simulink model "three_phase_solar_grid_SSC"  (R2025b)
settings: Solver=VariableStepAuto  StartTime=0.0  StopTime=0.8  RelTol=1e-6
libraries: ee_lib x15, nesl_utility x13, fl_lib x10, simulink x3, eeTransforms x2, eeSinusoidalMeasurementV2 x1
settings Model: SimulationMode=accelerator  Creator=a6039  LastModifiedBy=agarcian
settings SolverCC: AlgebraicLoopSolver=TrustRegion
settings DebuggingCC: UnconnectedInputMsg=warning  UnconnectedOutputMsg=warning  UnconnectedLineMsg=warning
settings ModelReferenceCC: EnableRefExpFcnMdlSchedulingChecks=on
settings RTWCC: GPUComputeCapability=3.5  DLArmComputeVersion=19.05

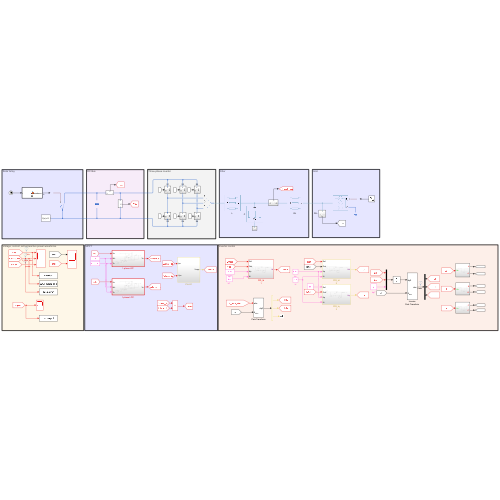
[thumbnail: Simulink's stored preview of the top-level diagram]
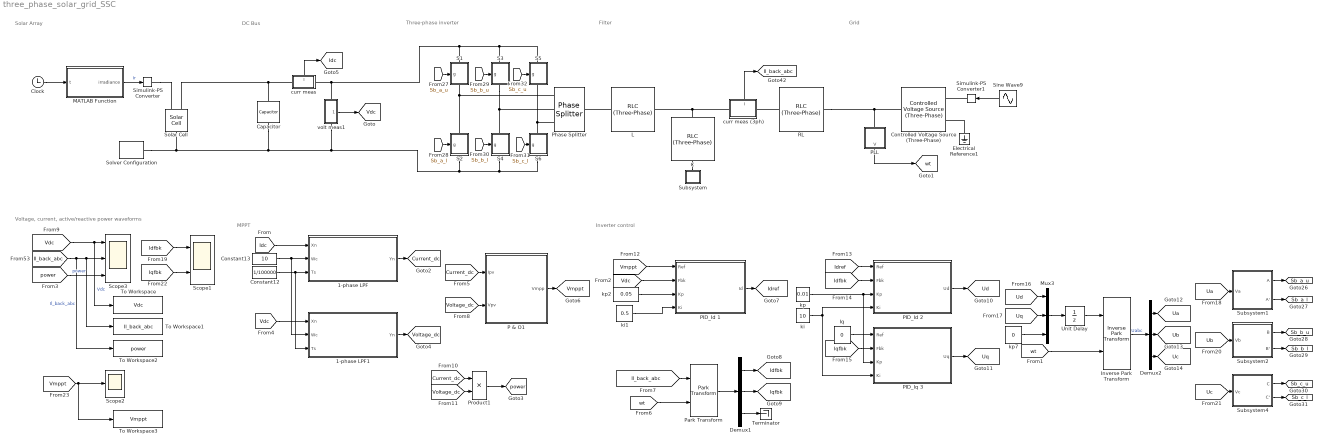
== system three_phase_solar_grid_SSC ==
  note: Filter
  note: Solar Array
  note: MPPT
  note: Three-phase inverter
  note: Inverter control
  note: Voltage, current, active/reactive power waveforms
  note: DC Bus
  note: Grid
  1-phase LPF : Subsystem  TreatAsAtomicUnit=on
  1-phase LPF1 : Subsystem  TreatAsAtomicUnit=on
  C : ee_lib/Passive/RLC Assemblies/RLC (Three-Phase)  port_option=ee.enum.threePhasePort.composite  component_structure=ee.enum.rlc.structure.C  R=1 Ohm  L=1e-3 H  C=1e-4 F  R_parasitic=0 Ohm  G_parasitic=0 1/Ohm  IL_specify=off  IL_priority=High  IL=[0, 0, 0] A  IL_nominal_specify=off  IL_nominal_value=1  IL_nominal_unit=A  VC_specify=off  VC_priority=High  VC=[0, 0, 0] V  VC_nominal_specify=off  VC_nominal_value=1  VC_nominal_unit=V
      settings: InternalSimscapePortConfiguration="{\"Bottom\":[],\"Left\":[{\"id\":\"N1\",\"label\":\"~1\",\"type\":\"foundation.electrical.three_phase\"}],\"Right\":[{\"id\":\"N2\",\"label\":\"~2\",\"type\":\"foundation.electrical.three_phase\"}],\"Top\":[]}"
  Capacitor : fl_lib/Electrical/Electrical Elements/Capacitor  c=1e-3 F  r=1e-8 Ohm  g=0 1/Ohm  i_specify=off  i_priority=None  i=0 A  i_nominal_specify=off  i_nominal_value=1  i_nominal_unit=A  v_specify=off  v_priority=None  v=0 V  v_nominal_specify=off  v_nominal_value=1  v_nominal_unit=V  vc_specify=off  vc_priority=High  vc=0 V  vc_nominal_specify=off  vc_nominal_value=1  vc_nominal_unit=V
  Clock : Clock
  Constant12 : Constant  Value=1/100000
  Constant13 : Constant  Value=10
  Controlled Voltage Source (Three-Phase) : ee_lib/Sources/Controlled Voltage Source (Three-Phase)  input_option=ee.enum.inputType.instantaneous  FRated=60 Hz
      settings: InternalSimscapePortConfiguration="{\"Bottom\":[],\"Left\":[{\"id\":\"S\",\"label\":\"S\",\"type\":\"input\"},{\"id\":\"n\",\"label\":\"n\",\"type\":\"foundation.electrical.electrical\"}],\"Right\":[{\"id\":\"N\",\"label\":\"~\",\"type\":\"foundation.electrical.three_phase\"}],\"Top\":[]}"
  Demux1 : Demux  Outputs=3
  Demux2 : Demux  Outputs=3
  Electrical Reference1 : fl_lib/Electrical/Electrical Elements/Electrical Reference
  Inverse Park Transform : eeTransforms/Inverse Park Transform  AxisAlignment=D-axis  PowerInvariant=off
      settings: LibrarySourceBlock=|
      | ee_sl_lib/Mathematical
      | Transforms/Inverse
      | Park Transform
  Iq : Constant  Value=0
  L : ee_lib/Passive/RLC Assemblies/RLC (Three-Phase)  port_option=ee.enum.threePhasePort.composite  component_structure=ee.enum.rlc.structure.L  R=1 Ohm  L=1e-3 H  C=1e-6 F  R_parasitic=0 Ohm  G_parasitic=0 1/Ohm  IL_specify=off  IL_priority=High  IL=[0, 0, 0] A  IL_nominal_specify=off  IL_nominal_value=1  IL_nominal_unit=A  VC_specify=off  VC_priority=High  VC=[0, 0, 0] V  VC_nominal_specify=off  VC_nominal_value=1  VC_nominal_unit=V
      settings: InternalSimscapePortConfiguration="{\"Bottom\":[],\"Left\":[{\"id\":\"N1\",\"label\":\"~1\",\"type\":\"foundation.electrical.three_phase\"}],\"Right\":[{\"id\":\"N2\",\"label\":\"~2\",\"type\":\"foundation.electrical.three_phase\"}],\"Top\":[]}"
  MATLAB Function : MATLAB Function  TreatAsAtomicUnit=on
  Mux3 : Mux  Inputs=3
  P & O1 : Subsystem
  PID_Id 1 : Subsystem
  PID_Id 2 : Subsystem
  PID_Iq 3 : Subsystem
  PLL : Subsystem
  Park Transform : eeTransforms/Park Transform  AxisAlignment=D-axis  PowerInvariant=off
      settings: LibrarySourceBlock=|
      | ee_sl_lib/Mathematical
      | Transforms/Park Transform
  Phase Splitter : ee_lib/Connectors & References/Phase Splitter
  Product1 : Product
  RL : ee_lib/Passive/RLC Assemblies/RLC (Three-Phase)  port_option=ee.enum.threePhasePort.composite  component_structure=ee.enum.rlc.structure.SeriesRL  R=0.1 Ohm  L=1e-9 H  C=1e-6 F  R_parasitic=0 Ohm  G_parasitic=0 1/Ohm  IL_specify=off  IL_priority=High  IL=[0, 0, 0] A  IL_nominal_specify=off  IL_nominal_value=1  IL_nominal_unit=A  VC_specify=off  VC_priority=High  VC=[0, 0, 0] V  VC_nominal_specify=off  VC_nominal_value=1  VC_nominal_unit=V
      settings: InternalSimscapePortConfiguration="{\"Bottom\":[],\"Left\":[{\"id\":\"N1\",\"label\":\"~1\",\"type\":\"foundation.electrical.three_phase\"}],\"Right\":[{\"id\":\"N2\",\"label\":\"~2\",\"type\":\"foundation.electrical.three_phase\"}],\"Top\":[]}"
  S1 : Subsystem
      settings: PortSchema="{\"entries\":[{\"content\":{\"sides\":[{\"content\":{\"connectorIds\":[\"In1\"]},\"type\":\"ConnectorPlacement.EquallySpacedRectSide\",\"uuid\":\"60fc8352-b056-4a1d-84e9-807da1ce3c88\"},{\"content\":{\"side\":\"RIGHT\"},\"type\":\"ConnectorPlacement.EquallySpacedRectSide\",\"uuid\":\"4f85bb6a-64c7-4bda-b651-7e84ba390faf\"},{\"content\":{\"connectorIds\":[\"LConn1\"],\"side\":\"TOP\"},\"type\":\"ConnectorPlacement.EquallySpacedRectSide\",\"uuid\":\"49a2dfe1-7dda-4371-a15a-7ad00d7eb6fd\"},{\"content\":{\"connectorIds\":[\"RConn1\"],\"side\":\"BOTTOM\"},\"type\":\"ConnectorPlacement.EquallySpacedRectSide\",\"uuid\":\"2b076144-f23a-4c54-b109-69957c2c042c\"}]},\"type\":\"ConnectorPlacement.EquallySpacedConnector\",\"uuid\":\"c494b7b1-a248-4760-aec7-aedba1239c75\"}],\"packageUris\":[\"http://schema.mathworks.com/mf0/Connector/R2020b\"],\"version\":\"1.0\"}"
  S2 : Subsystem
      settings: PortSchema="{\"entries\":[{\"content\":{\"sides\":[{\"content\":{\"connectorIds\":[\"In1\"]},\"type\":\"ConnectorPlacement.EquallySpacedRectSide\",\"uuid\":\"60fc8352-b056-4a1d-84e9-807da1ce3c88\"},{\"content\":{\"side\":\"RIGHT\"},\"type\":\"ConnectorPlacement.EquallySpacedRectSide\",\"uuid\":\"4f85bb6a-64c7-4bda-b651-7e84ba390faf\"},{\"content\":{\"connectorIds\":[\"LConn1\"],\"side\":\"TOP\"},\"type\":\"ConnectorPlacement.EquallySpacedRectSide\",\"uuid\":\"49a2dfe1-7dda-4371-a15a-7ad00d7eb6fd\"},{\"content\":{\"connectorIds\":[\"RConn1\"],\"side\":\"BOTTOM\"},\"type\":\"ConnectorPlacement.EquallySpacedRectSide\",\"uuid\":\"2b076144-f23a-4c54-b109-69957c2c042c\"}]},\"type\":\"ConnectorPlacement.EquallySpacedConnector\",\"uuid\":\"c494b7b1-a248-4760-aec7-aedba1239c75\"}],\"packageUris\":[\"http://schema.mathworks.com/mf0/Connector/R2020b\"],\"version\":\"1.0\"}"
  S3 : Subsystem
      settings: PortSchema="{\"entries\":[{\"content\":{\"sides\":[{\"content\":{\"connectorIds\":[\"In1\"]},\"type\":\"ConnectorPlacement.EquallySpacedRectSide\",\"uuid\":\"60fc8352-b056-4a1d-84e9-807da1ce3c88\"},{\"content\":{\"side\":\"RIGHT\"},\"type\":\"ConnectorPlacement.EquallySpacedRectSide\",\"uuid\":\"4f85bb6a-64c7-4bda-b651-7e84ba390faf\"},{\"content\":{\"connectorIds\":[\"LConn1\"],\"side\":\"TOP\"},\"type\":\"ConnectorPlacement.EquallySpacedRectSide\",\"uuid\":\"49a2dfe1-7dda-4371-a15a-7ad00d7eb6fd\"},{\"content\":{\"connectorIds\":[\"RConn1\"],\"side\":\"BOTTOM\"},\"type\":\"ConnectorPlacement.EquallySpacedRectSide\",\"uuid\":\"2b076144-f23a-4c54-b109-69957c2c042c\"}]},\"type\":\"ConnectorPlacement.EquallySpacedConnector\",\"uuid\":\"c494b7b1-a248-4760-aec7-aedba1239c75\"}],\"packageUris\":[\"http://schema.mathworks.com/mf0/Connector/R2020b\"],\"version\":\"1.0\"}"
  S4 : Subsystem
      settings: PortSchema="{\"entries\":[{\"content\":{\"sides\":[{\"content\":{\"connectorIds\":[\"In1\"]},\"type\":\"ConnectorPlacement.EquallySpacedRectSide\",\"uuid\":\"60fc8352-b056-4a1d-84e9-807da1ce3c88\"},{\"content\":{\"side\":\"RIGHT\"},\"type\":\"ConnectorPlacement.EquallySpacedRectSide\",\"uuid\":\"4f85bb6a-64c7-4bda-b651-7e84ba390faf\"},{\"content\":{\"connectorIds\":[\"LConn1\"],\"side\":\"TOP\"},\"type\":\"ConnectorPlacement.EquallySpacedRectSide\",\"uuid\":\"49a2dfe1-7dda-4371-a15a-7ad00d7eb6fd\"},{\"content\":{\"connectorIds\":[\"RConn1\"],\"side\":\"BOTTOM\"},\"type\":\"ConnectorPlacement.EquallySpacedRectSide\",\"uuid\":\"2b076144-f23a-4c54-b109-69957c2c042c\"}]},\"type\":\"ConnectorPlacement.EquallySpacedConnector\",\"uuid\":\"c494b7b1-a248-4760-aec7-aedba1239c75\"}],\"packageUris\":[\"http://schema.mathworks.com/mf0/Connector/R2020b\"],\"version\":\"1.0\"}"
  S5 : Subsystem
      settings: PortSchema="{\"entries\":[{\"content\":{\"sides\":[{\"content\":{\"connectorIds\":[\"In1\"]},\"type\":\"ConnectorPlacement.EquallySpacedRectSide\",\"uuid\":\"60fc8352-b056-4a1d-84e9-807da1ce3c88\"},{\"content\":{\"side\":\"RIGHT\"},\"type\":\"ConnectorPlacement.EquallySpacedRectSide\",\"uuid\":\"4f85bb6a-64c7-4bda-b651-7e84ba390faf\"},{\"content\":{\"connectorIds\":[\"LConn1\"],\"side\":\"TOP\"},\"type\":\"ConnectorPlacement.EquallySpacedRectSide\",\"uuid\":\"49a2dfe1-7dda-4371-a15a-7ad00d7eb6fd\"},{\"content\":{\"connectorIds\":[\"RConn1\"],\"side\":\"BOTTOM\"},\"type\":\"ConnectorPlacement.EquallySpacedRectSide\",\"uuid\":\"2b076144-f23a-4c54-b109-69957c2c042c\"}]},\"type\":\"ConnectorPlacement.EquallySpacedConnector\",\"uuid\":\"c494b7b1-a248-4760-aec7-aedba1239c75\"}],\"packageUris\":[\"http://schema.mathworks.com/mf0/Connector/R2020b\"],\"version\":\"1.0\"}"
  S6 : Subsystem
      settings: PortSchema="{\"entries\":[{\"content\":{\"sides\":[{\"content\":{\"connectorIds\":[\"In1\"]},\"type\":\"ConnectorPlacement.EquallySpacedRectSide\",\"uuid\":\"60fc8352-b056-4a1d-84e9-807da1ce3c88\"},{\"content\":{\"side\":\"RIGHT\"},\"type\":\"ConnectorPlacement.EquallySpacedRectSide\",\"uuid\":\"4f85bb6a-64c7-4bda-b651-7e84ba390faf\"},{\"content\":{\"connectorIds\":[\"LConn1\"],\"side\":\"TOP\"},\"type\":\"ConnectorPlacement.EquallySpacedRectSide\",\"uuid\":\"49a2dfe1-7dda-4371-a15a-7ad00d7eb6fd\"},{\"content\":{\"connectorIds\":[\"RConn1\"],\"side\":\"BOTTOM\"},\"type\":\"ConnectorPlacement.EquallySpacedRectSide\",\"uuid\":\"2b076144-f23a-4c54-b109-69957c2c042c\"}]},\"type\":\"ConnectorPlacement.EquallySpacedConnector\",\"uuid\":\"c494b7b1-a248-4760-aec7-aedba1239c75\"}],\"packageUris\":[\"http://schema.mathworks.com/mf0/Connector/R2020b\"],\"version\":\"1.0\"}"
  Scope1 : Scope  NumInputPorts=2
      settings: ActiveDisplayYMinimum=-149.18655  ActiveDisplayYMaximum=893.7115
  Scope2 : Scope
      settings: ActiveDisplayYMinimum=356.99125  ActiveDisplayYMaximum=407.77875  DataLoggingVariableName=ScopeData2
  Scope3 : Scope  NumInputPorts=3
      settings: ActiveDisplayYMinimum=-56.521329530696754  ActiveDisplayYMaximum=508.69198645627091  DataLoggingVariableName=ScopeData3
  Simulink-PS Converter : nesl_utility/Simulink-PS Converter  PhysicalDomain=network_engine_domain  SubClassName=ps_input  LeftPortType=input  RightPortType=output  PseudoPeriodic=off  Frequencies=[]  NoiseDistribution=none  NoiseParameters=[]  Unit=1  AffineConversion=off  FilteringAndDerivatives=provide  SimscapeFilterOrder=1  InputFilterTimeConstant=0.001  UdotUserProvided=0
  Simulink-PS Converter1 : nesl_utility/Simulink-PS Converter  PhysicalDomain=network_engine_domain  SubClassName=ps_input  LeftPortType=input  RightPortType=output  PseudoPeriodic=off  Frequencies=[]  NoiseDistribution=none  NoiseParameters=[]  Unit=1  AffineConversion=off  FilteringAndDerivatives=provide  SimscapeFilterOrder=1  InputFilterTimeConstant=0.001  UdotUserProvided=0
  Sine Wave9 : Sin  Amplitude=169.7  Frequency=60*2*pi  Phase=[0 -1 1]*2*pi/3  SampleTime=0
  Solar Cell : ee_lib/Sources/Solar Cell  prm=ee.enum.sources.solar_cell_prm.datasheet  Isc=5.17 A  Voc=43.99/72 V  Is=1e-6 A  Is2=0 A  Iph=7.34 A  Ir0=1000 W/m^2  ec=1.5  N2=2  Rs=0 Ohm  Rp=inf Ohm  N_series=10*72  N_parallel=40  TIPH1=0 1/K  EG=1.11 eV  TXIS1=3  TXIS2=3  TRS1=0  TRP1=0  Tmeas=25 degC  TFIXED=25 degC  thermal_mass=100 J/K  initial_temperature=25 degC
  Solver Configuration : nesl_utility/Solver Configuration  PhysicalDomain=network_engine_domain  SubClassName=solver  LeftPortType=input  RightPortType=generic  Tones=[]  Harmonics=[]  SimulateNoise=off  Profile=off  UseLocalSampling=off  EnableSwitchedLinearOptims=on  FrequencyDomain=off  UseCCode=off  RelTol=0.001  AbsTol=0.001  MinStep=1e-09  ToWorkspace=off  RevertToSquareIcSolve=off  NumHomotopyIterations=100  PhasorMode=off  PhasorModeNumHarmonics=1  ConsistencySolver=NEWTON_XTOL_AFTER_FTOL  IndexReductionMethod=DerivativeReplacement  DoDC=off  ResidualTolerance=1e-09  ConsistencyTolSource=GLOBAL  ConsistencyAbsTol=0.001  ConsistencyRelTol=0.001  ConsistencyTolFactor=0.001  UseLocalSolver=on  LocalSolverChoice=NE_BACKWARD_EULER_ADVANCER  ResolveIndetEquations=off  FunctionEvalNumThread=1  LocalSolverSampleTime=1e-7  DoFixedCost=on  MaxNonlinIter=2  MaxModeIter=2  ComputeImpulses=off  ImpulseIterations=2  LinearAlgebra=auto  LinearAlgebraNumThread=0  EquationFormulation=NE_TIME_EF  DelaysMemoryBudget=1024  AutomaticFiltering=off  FilteringTimeConstant=0.001  PartitionStorageMethod=AS_NEEDED  PartitionMemoryBudget=1024  PartitionMethod=FAST  MultibodyUseLocalSolver=off  MultibodyLocalSolverChoice=ODE1  MultibodyLocalSolverSampleTime=0.001
  Subsystem : Subsystem
  Subsystem1 : Subsystem
  Subsystem2 : Subsystem
  Subsystem4 : Subsystem
  Terminator : Terminator
  To Workspace : ToWorkspace  VariableName=Vdc  SaveFormat=Structure With Time  SampleTime=-1
  To Workspace1 : ToWorkspace  VariableName=Il_back_abc  SaveFormat=Structure With Time  SampleTime=-1
  To Workspace2 : ToWorkspace  VariableName=power  SaveFormat=Structure With Time  SampleTime=-1
  To Workspace3 : ToWorkspace  VariableName=Vmppt  SaveFormat=Structure With Time  SampleTime=-1
  Unit Delay : UnitDelay  SampleTime=-1  HasFrameUpgradeWarning=on
  curr meas : Subsystem
      settings: PortSchema="{\"entries\":[{\"content\":{\"sides\":[{\"content\":{\"connectorIds\":[\"LConn1\"]},\"type\":\"ConnectorPlacement.EquallySpacedRectSide\",\"uuid\":\"624dd8c9-1efa-425a-b23f-9e7d392e4567\"},{\"content\":{\"connectorIds\":[\"RConn1\"],\"side\":\"RIGHT\"},\"type\":\"ConnectorPlacement.EquallySpacedRectSide\",\"uuid\":\"c564bb74-22a6-4c48-884d-57ae53c7e586\"},{\"content\":{\"connectorIds\":[\"Out1\"],\"side\":\"TOP\"},\"type\":\"ConnectorPlacement.EquallySpacedRectSide\",\"uuid\":\"df3a0756-8bf4-4498-aa4e-0bb1b4f3eded\"}]},\"type\":\"ConnectorPlacement.EquallySpacedConnector\",\"uuid\":\"9eff73ec-b3ab-492c-96fa-8ca694a66385\"}],\"packageUris\":[\"http://schema.mathworks.com/mf0/Connector/R2020b\"],\"version\":\"1.0\"}"
  curr meas (3ph) : Subsystem
      settings: PortSchema="{\"entries\":[{\"content\":{\"sides\":[{\"content\":{\"connectorIds\":[\"LConn1\"]},\"type\":\"ConnectorPlacement.EquallySpacedRectSide\",\"uuid\":\"624dd8c9-1efa-425a-b23f-9e7d392e4567\"},{\"content\":{\"connectorIds\":[\"RConn1\"],\"side\":\"RIGHT\"},\"type\":\"ConnectorPlacement.EquallySpacedRectSide\",\"uuid\":\"c564bb74-22a6-4c48-884d-57ae53c7e586\"},{\"content\":{\"connectorIds\":[\"Out1\"],\"side\":\"TOP\"},\"type\":\"ConnectorPlacement.EquallySpacedRectSide\",\"uuid\":\"df3a0756-8bf4-4498-aa4e-0bb1b4f3eded\"}]},\"type\":\"ConnectorPlacement.EquallySpacedConnector\",\"uuid\":\"9eff73ec-b3ab-492c-96fa-8ca694a66385\"}],\"packageUris\":[\"http://schema.mathworks.com/mf0/Connector/R2020b\"],\"version\":\"1.0\"}"
  ki : Constant  Value=10
  ki1 : Constant  Value=0.5
  kp : Constant  Value=0.01
  kp2 : Constant  Value=0.05
  kp7 : Constant  Value=0
  volt meas1 : Subsystem
      settings: PortSchema="{\"entries\":[{\"content\":{\"sides\":[{\"content\":{},\"type\":\"ConnectorPlacement.EquallySpacedRectSide\",\"uuid\":\"624dd8c9-1efa-425a-b23f-9e7d392e4567\"},{\"content\":{\"connectorIds\":[\"Out1\"],\"side\":\"RIGHT\"},\"type\":\"ConnectorPlacement.EquallySpacedRectSide\",\"uuid\":\"c564bb74-22a6-4c48-884d-57ae53c7e586\"},{\"content\":{\"connectorIds\":[\"LConn1\"],\"side\":\"TOP\"},\"type\":\"ConnectorPlacement.EquallySpacedRectSide\",\"uuid\":\"df3a0756-8bf4-4498-aa4e-0bb1b4f3eded\"},{\"content\":{\"connectorIds\":[\"RConn1\"],\"side\":\"BOTTOM\"},\"type\":\"ConnectorPlacement.EquallySpacedRectSide\",\"uuid\":\"6b8e9540-8d6f-4bd3-bf1f-20eb25478a8e\"}]},\"type\":\"ConnectorPlacement.EquallySpacedConnector\",\"uuid\":\"9eff73ec-b3ab-492c-96fa-8ca694a66385\"}],\"packageUris\":[\"http://schema.mathworks.com/mf0/Connector/R2020b\"],\"version\":\"1.0\"}"
  tag scope: Current_dc=global, Idc=global, Idfbk=global, Idref=global, Il_back_abc=global, Iqfbk=global, Sb_a_l=global, Sb_a_u=global, Sb_b_l=global, Sb_b_u=global, Sb_c_l=global, Sb_c_u=global, Ua=global, Ub=global, Uc=global, Ud=global, Uq=global, Vdc=global, Vmppt=global, Voltage_dc=global, power=global, wt=global
  wires:
  [Il_back_abc] -> To Workspace2/1, To Workspace1/1, Scope3/2  "Il_back_abc"
  Iq/1 -> PID_Iq 3/1(Ref)
  Park Transform/1 -> Demux1/1
  [wt] -> Inverse Park Transform/2
  kp/1 -> PID_Iq 3/3(Kp), PID_Id 2/3(Kp)
  ki/1 -> PID_Id 2/4(Ki), PID_Iq 3/4(Ki)
  Mux3/1 -> Unit Delay/1
  [wt] -> Park Transform/2
  Inverse Park Transform/1 -> Demux2/1  "Uabc"
  [Il_back_abc] -> Park Transform/1
  [Sb_a_u] -> S1/1(g)
  [Sb_b_u] -> S3/1(g)
  [Sb_c_u] -> S5/1(g)
  [Sb_a_l] -> S2/1(g)
  [Sb_b_l] -> S4/1(g)
  [Sb_c_l] -> S6/1(g)
  volt meas1/1(V) -> [Vdc]
  [Vdc] -> PID_Id 1/2(Fbk)
  kp2/1 -> PID_Id 1/3(Kp)
  ki1/1 -> PID_Id 1/4(Ki)
  Constant12/1 -> 1-phase LPF1/3(Ts), 1-phase LPF/3(Ts)
  Constant13/1 -> 1-phase LPF1/2(Wc), 1-phase LPF/2(Wc)
  [Idc] -> 1-phase LPF/1(Xn)
  [Vdc] -> 1-phase LPF1/1(Xn)
  Subsystem1/1(A) -> [Sb_a_u]
  Subsystem1/2(A') -> [Sb_a_l]
  Subsystem2/1(B) -> [Sb_b_u]
  Subsystem2/2(B') -> [Sb_b_l]
  Subsystem4/1(C) -> [Sb_c_u]
  Subsystem4/2(C') -> [Sb_c_l]
  kp7/1 -> Mux3/3
  [Vdc] -> To Workspace/1, Scope3/1  "Vdc"
  [power] -> Scope3/3  "power"
  Product1/1 -> [power]
  Clock/1 -> MATLAB Function/1(t)
  1-phase LPF/1(Yn) -> [Current_dc]
  1-phase LPF1/1(Yn) -> [Voltage_dc]
  [Current_dc] -> P & O1/1(Ipv)
  [Voltage_dc] -> P & O1/2(Vpv)
  [Current_dc] -> Product1/1
  [Voltage_dc] -> Product1/2
  P & O1/1(Vmpp) -> [Vmppt]
  [Vmppt] -> PID_Id 1/1(Ref)
  PID_Id 1/1(Id) -> [Idref]
  [Idref] -> PID_Id 2/1(Ref)
  Demux1/1 -> [Idfbk]
  Demux1/2 -> [Iqfbk]
  [Idfbk] -> PID_Id 2/2(Fbk)
  [Iqfbk] -> PID_Iq 3/2(Fbk)
  PID_Id 2/1(Ud) -> [Ud]
  PID_Iq 3/1(Uq) -> [Uq]
  [Ud] -> Mux3/1
  [Uq] -> Mux3/2
  Demux2/1 -> [Ua]
  Demux2/2 -> [Ub]
  Demux2/3 -> [Uc]
  [Ua] -> Subsystem1/1(Va)
  [Ub] -> Subsystem2/1(Vb)
  [Uc] -> Subsystem4/1(Vc)
  [Idfbk] -> Scope1/1
  [Iqfbk] -> Scope1/2
  [Vmppt] -> To Workspace3/1, Scope2/1
  MATLAB Function/1(irradiance) -> Simulink-PS Converter/1  "Ir"
  curr meas/1(I) -> [Idc]
  curr meas (3ph)/1(I) -> [Il_back_abc]
  Sine Wave9/1 -> Simulink-PS Converter1/1
  Unit Delay/1 -> Inverse Park Transform/1
  Demux1/3 -> Terminator/1
  PLL/1(V) -> [wt]
  connections:
  volt meas1/LConn1 -- S5/LConn1 -- S3/LConn1 -- S1/LConn1 -- curr meas/RConn1
  Phase Splitter/RConn2 -- S3/RConn1 -- S4/LConn1
  Solver Configuration/RConn1 -- S6/RConn1 -- S4/RConn1 -- S2/RConn1 -- volt meas1/RConn1 -- Capacitor/RConn1 -- Solar Cell/RConn1
  Simulink-PS Converter/RConn1 -- Solar Cell/LConn1
  Phase Splitter/RConn1 -- S2/LConn1 -- S1/RConn1
  L/LConn1 -- Phase Splitter/LConn1
  C/LConn1 -- curr meas (3ph)/LConn1 -- L/RConn1
  RL/LConn1 -- curr meas (3ph)/RConn1
  RL/RConn1 -- Controlled Voltage Source (Three-Phase)/RConn1 -- PLL/LConn1
  Simulink-PS Converter1/RConn1 -- Controlled Voltage Source (Three-Phase)/LConn1
  Electrical Reference1/LConn1 -- Controlled Voltage Source (Three-Phase)/LConn2
  S6/LConn1 -- Phase Splitter/RConn3 -- S5/RConn1
  C/RConn1 -- Subsystem/LConn1
  Capacitor/LConn1 -- Solar Cell/LConn2 -- curr meas/LConn1

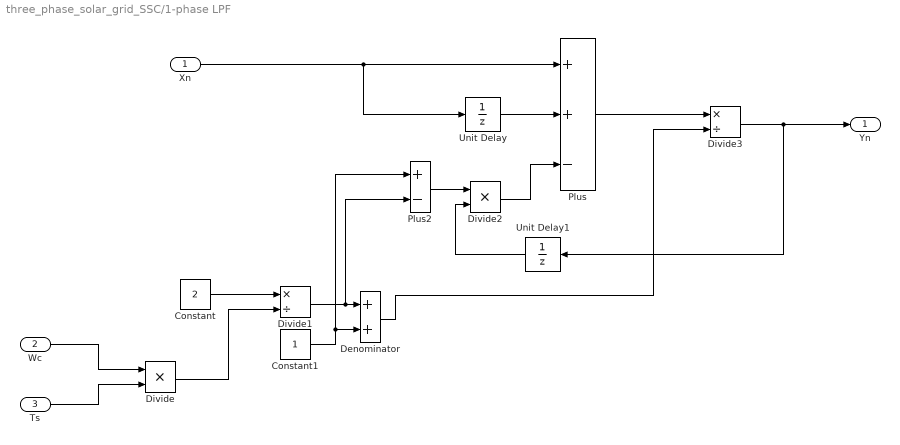
== system three_phase_solar_grid_SSC/1-phase LPF ==
  Xn : Inport
  Wc : Inport  Port=2
  Ts : Inport  Port=3
  Constant : Constant  Value=2
  Constant1 : Constant
  Denominator : Sum
  Divide : Product  Inputs=**
  Divide1 : Product  Inputs=*/
  Divide2 : Product  Inputs=**
  Divide3 : Product  Inputs=*/
  Plus : Sum  Inputs=++-
  Plus2 : Sum  Inputs=+-
  Unit Delay : UnitDelay  SampleTime=-1  HasFrameUpgradeWarning=on
  Unit Delay1 : UnitDelay  SampleTime=-1  HasFrameUpgradeWarning=on
  Yn : Outport
  wires:
  Xn/1 -> Unit Delay/1, Plus/1
  Unit Delay/1 -> Plus/2
  Wc/1 -> Divide/1
  Ts/1 -> Divide/2
  Divide/1 -> Divide1/2
  Constant/1 -> Divide1/1
  Divide1/1 -> Plus2/2, Denominator/1
  Constant1/1 -> Plus2/1, Denominator/2
  Plus2/1 -> Divide2/1
  Unit Delay1/1 -> Divide2/2
  Plus/1 -> Divide3/1
  Denominator/1 -> Divide3/2
  Divide3/1 -> Unit Delay1/1, Yn/1
  Divide2/1 -> Plus/3

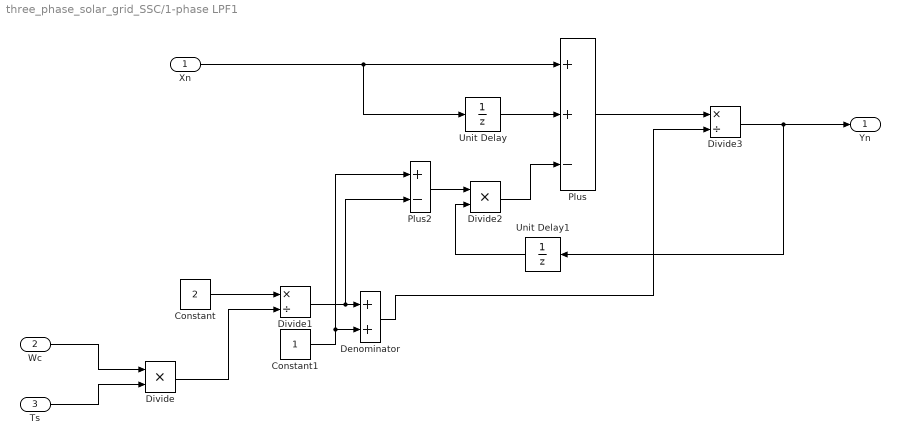
== system three_phase_solar_grid_SSC/1-phase LPF1 ==
  Xn : Inport
  Wc : Inport  Port=2
  Ts : Inport  Port=3
  Constant : Constant  Value=2
  Constant1 : Constant
  Denominator : Sum
  Divide : Product  Inputs=**
  Divide1 : Product  Inputs=*/
  Divide2 : Product  Inputs=**
  Divide3 : Product  Inputs=*/
  Plus : Sum  Inputs=++-
  Plus2 : Sum  Inputs=+-
  Unit Delay : UnitDelay  SampleTime=-1  HasFrameUpgradeWarning=on
  Unit Delay1 : UnitDelay  SampleTime=-1  HasFrameUpgradeWarning=on
  Yn : Outport
  wires:
  Xn/1 -> Unit Delay/1, Plus/1
  Unit Delay/1 -> Plus/2
  Wc/1 -> Divide/1
  Ts/1 -> Divide/2
  Divide/1 -> Divide1/2
  Constant/1 -> Divide1/1
  Divide1/1 -> Plus2/2, Denominator/1
  Constant1/1 -> Plus2/1, Denominator/2
  Plus2/1 -> Divide2/1
  Unit Delay1/1 -> Divide2/2
  Plus/1 -> Divide3/1
  Denominator/1 -> Divide3/2
  Divide3/1 -> Unit Delay1/1, Yn/1
  Divide2/1 -> Plus/3

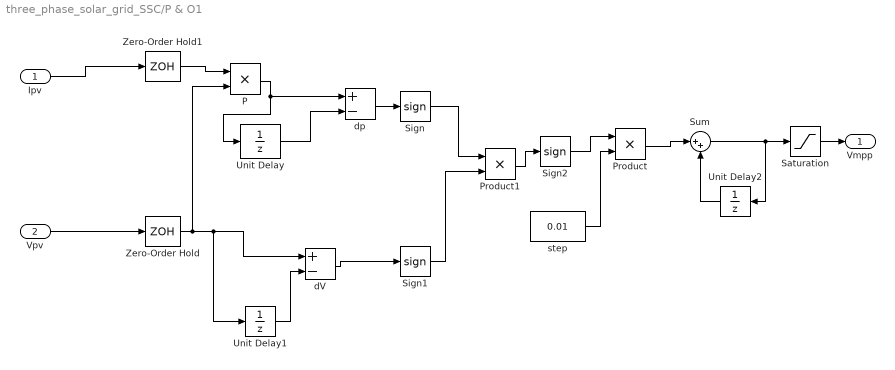
== system three_phase_solar_grid_SSC/P & O1 ==
  Ipv : Inport
  Vpv : Inport  Port=2
  P : Product  RndMeth=Zero
  Product : Product  RndMeth=Zero
  Product1 : Product  RndMeth=Zero
  Saturation : Saturate  UpperLimit=450  LowerLimit=0  LinearizeAsGain=off  ZeroCross=off
  Sign : Signum
  Sign1 : Signum
  Sign2 : Signum
  Sum : Sum  Inputs=|++
  Unit Delay : UnitDelay  SampleTime=-1  HasFrameUpgradeWarning=on
  Unit Delay1 : UnitDelay  SampleTime=-1  HasFrameUpgradeWarning=on
  Unit Delay2 : UnitDelay  InitialCondition=400  SampleTime=-1  HasFrameUpgradeWarning=on
  Zero-Order Hold : ZeroOrderHold  SampleTime=1/100000
  Zero-Order Hold1 : ZeroOrderHold  SampleTime=1/100000
  dV : Sum  Inputs=+-
  dp : Sum  Inputs=+-
  step : Constant  Value=0.01  SampleTime=1/100000
  Vmpp : Outport
  wires:
  Unit Delay1/1 -> dV/2
  Unit Delay/1 -> dp/2
  dV/1 -> Sign1/1
  step/1 -> Product/2
  Product/1 -> Sum/1
  Sign/1 -> Product1/1
  Sign1/1 -> Product1/2
  Product1/1 -> Sign2/1
  Ipv/1 -> Zero-Order Hold1/1
  Vpv/1 -> Zero-Order Hold/1
  P/1 -> Unit Delay/1, dp/1
  dp/1 -> Sign/1
  Sign2/1 -> Product/1
  Sum/1 -> Saturation/1, Unit Delay2/1
  Unit Delay2/1 -> Sum/2
  Zero-Order Hold/1 -> P/2, Unit Delay1/1, dV/1
  Zero-Order Hold1/1 -> P/1
  Saturation/1 -> Vmpp/1

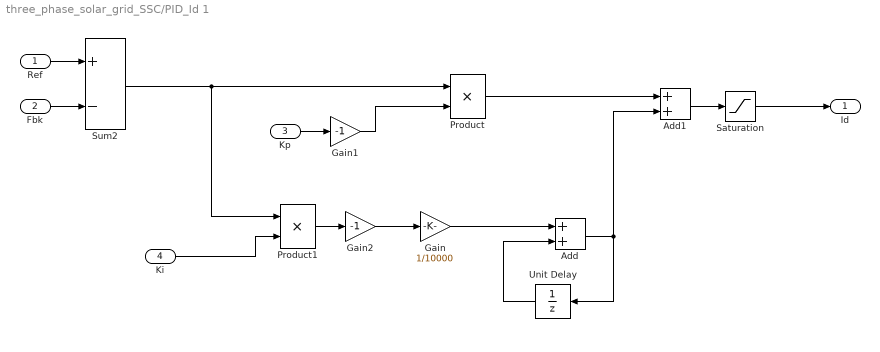
== system three_phase_solar_grid_SSC/PID_Id 1 ==
  Ref : Inport
  Fbk : Inport  Port=2
  Kp : Inport  Port=3
  Ki : Inport  Port=4
  Add : Sum
  Add1 : Sum
  Gain : Gain  Gain=1/10000
  Gain1 : Gain  Gain=-1
  Gain2 : Gain  Gain=-1
  Product : Product  OutDataTypeStr=Inherit: Same as first input
  Product1 : Product  OutDataTypeStr=Inherit: Same as first input
  Saturation : Saturate  UpperLimit=1000  LowerLimit=0  LinearizeAsGain=off  ZeroCross=off
  Sum2 : Sum  Inputs=+-
  Unit Delay : UnitDelay  SampleTime=-1  HasFrameUpgradeWarning=on
  Id : Outport
  wires:
  Sum2/1 -> Product1/1, Product/1
  Fbk/1 -> Sum2/2
  Ref/1 -> Sum2/1
  Product1/1 -> Gain2/1
  Add/1 -> Unit Delay/1, Add1/2
  Product/1 -> Add1/1
  Gain/1 -> Add/1
  Unit Delay/1 -> Add/2
  Kp/1 -> Gain1/1
  Ki/1 -> Product1/2
  Gain1/1 -> Product/2
  Gain2/1 -> Gain/1
  Add1/1 -> Saturation/1
  Saturation/1 -> Id/1

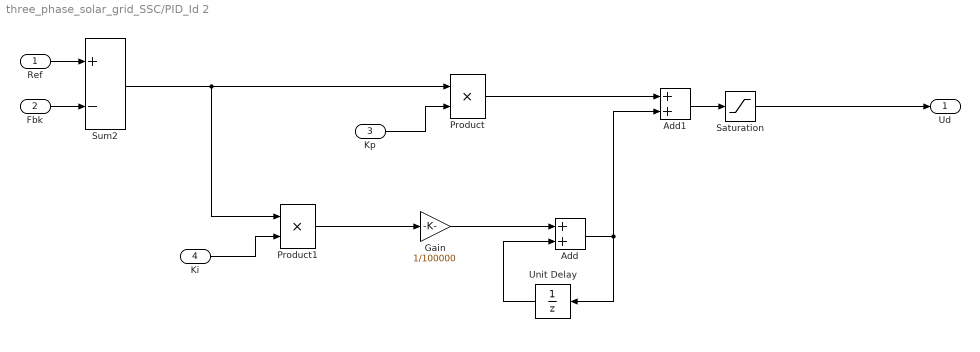
== system three_phase_solar_grid_SSC/PID_Id 2 ==
  Ref : Inport
  Fbk : Inport  Port=2
  Kp : Inport  Port=3
  Ki : Inport  Port=4
  Add : Sum
  Add1 : Sum
  Gain : Gain  Gain=1/100000
  Product : Product  OutDataTypeStr=Inherit: Same as first input
  Product1 : Product  OutDataTypeStr=Inherit: Same as first input
  Saturation : Saturate  UpperLimit=500  LowerLimit=-500  LinearizeAsGain=off  ZeroCross=off
  Sum2 : Sum  Inputs=+-
  Unit Delay : UnitDelay  InitialCondition=400  SampleTime=-1  HasFrameUpgradeWarning=on
  Ud : Outport
  wires:
  Add1/1 -> Saturation/1
  Sum2/1 -> Product1/1, Product/1
  Fbk/1 -> Sum2/2
  Ref/1 -> Sum2/1
  Kp/1 -> Product/2
  Ki/1 -> Product1/2
  Product1/1 -> Gain/1
  Add/1 -> Unit Delay/1, Add1/2
  Product/1 -> Add1/1
  Saturation/1 -> Ud/1
  Gain/1 -> Add/1
  Unit Delay/1 -> Add/2

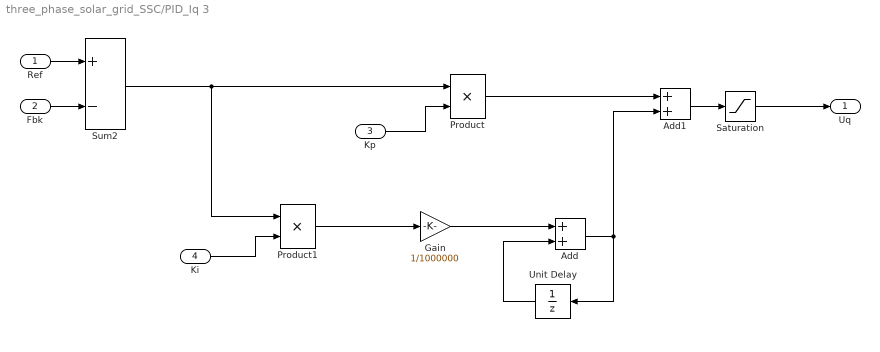
== system three_phase_solar_grid_SSC/PID_Iq 3 ==
  Ref : Inport
  Fbk : Inport  Port=2
  Kp : Inport  Port=3
  Ki : Inport  Port=4
  Add : Sum
  Add1 : Sum
  Gain : Gain  Gain=1/1000000
  Product : Product  OutDataTypeStr=Inherit: Same as first input
  Product1 : Product  OutDataTypeStr=Inherit: Same as first input
  Saturation : Saturate  UpperLimit=500  LowerLimit=-500  LinearizeAsGain=off  ZeroCross=off
  Sum2 : Sum  Inputs=+-
  Unit Delay : UnitDelay  SampleTime=-1  HasFrameUpgradeWarning=on
  Uq : Outport
  wires:
  Add1/1 -> Saturation/1
  Sum2/1 -> Product1/1, Product/1
  Fbk/1 -> Sum2/2
  Ref/1 -> Sum2/1
  Kp/1 -> Product/2
  Ki/1 -> Product1/2
  Product1/1 -> Gain/1
  Add/1 -> Unit Delay/1, Add1/2
  Product/1 -> Add1/1
  Gain/1 -> Add/1
  Unit Delay/1 -> Add/2
  Saturation/1 -> Uq/1

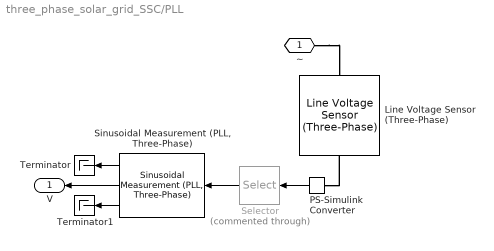
== system three_phase_solar_grid_SSC/PLL ==
  Line Voltage Sensor (Three-Phase) : ee_lib/Sensors & Transducers/Line Voltage Sensor (Three-Phase)
  PS-Simulink Converter : nesl_utility/PS-Simulink Converter  PhysicalDomain=network_engine_domain  SubClassName=ps_output  LeftPortType=input  RightPortType=output  PseudoPeriodic=off  Frequencies=[]  VectorFormat=inherit  Unit=inherit  AffineConversion=off
  Selector : Selector  Commented=through  InputPortWidth=3  IndexOptions=Index vector (dialog)  Indices=1  OutputSizes=1
  "Sinusoidal Measurement (PLL, Three-Phase)" : eeSinusoidalMeasurementV2/Sinusoidal Measurement (PLL, Three-Phase)  InputFilter=on  InputNormalization=off  Kp_LF=400  Ki_LF=20000  F0=60  Theta0=0  Ts=-1
      settings: LibrarySourceBlock=|
      | ee_sl_lib/Measurements/Sinusoidal Measurement
      | (PLL, Three-Phase)
  Terminator : Terminator
  Terminator1 : Terminator
  ~ : PMIOPort  Side=Left
  V : Outport
  wires:
  PS-Simulink Converter/1 -> Selector/1
  Selector/1 -> "Sinusoidal Measurement (PLL, Three-Phase)"/1
  "Sinusoidal Measurement (PLL, Three-Phase)"/1 -> Terminator/1
  "Sinusoidal Measurement (PLL, Three-Phase)"/3 -> Terminator1/1
  "Sinusoidal Measurement (PLL, Three-Phase)"/2 -> V/1
  connections:
  PS-Simulink Converter/LConn1 -- Line Voltage Sensor (Three-Phase)/RConn1
  ~/RConn1 -- Line Voltage Sensor (Three-Phase)/LConn1

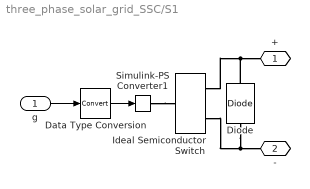
== system three_phase_solar_grid_SSC/S1 ==
  g : Inport
  Data Type Conversion : DataTypeConversion  SaturateOnIntegerOverflow=off  RndMeth=Floor
  Diode : fl_lib/Electrical/Electrical Elements/Diode  Vf=1e-3 V  Ron=0.01 Ohm  Goff=1e-5 1/Ohm  i_specify=off  i_priority=None  i=0 A  i_nominal_specify=off  i_nominal_value=1  i_nominal_unit=A  v_specify=off  v_priority=None  v=0 V  v_nominal_specify=off  v_nominal_value=1  v_nominal_unit=V
  Ideal Semiconductor Switch : ee_lib/Semiconductors & Converters/Ideal Semiconductor Switch  port_option=ee.enum.controlport.ps  Ron=0.1 Ohm  Goff=1e-5 1/Ohm  Vth=0.5 V  diode_param=ee.enum.semiconductors.protectionDiode.external  diode_Vf=1e-3 V  diode_Ron=0.01 Ohm  diode_Goff=1e-5 1/Ohm  diode_C=50e-9 F  diode_iRM=-235 A  diode_iF=300 A  diode_idot=-50 A/us  diode_trr_param=ee.enum.converters.diodetrr.trr_factor  diode_trr_factor=3  diode_trr=15 us  diode_Qrr=1500 s*uA
  Simulink-PS Converter1 : nesl_utility/Simulink-PS Converter  PhysicalDomain=network_engine_domain  SubClassName=ps_input  LeftPortType=input  RightPortType=output  PseudoPeriodic=off  Frequencies=[]  NoiseDistribution=none  NoiseParameters=[]  Unit=1  AffineConversion=off  FilteringAndDerivatives=provide  SimscapeFilterOrder=1  InputFilterTimeConstant=0.001  UdotUserProvided=0
  + : PMIOPort  Side=Left
  - : PMIOPort  Port=2  Side=Right
  wires:
  g/1 -> Data Type Conversion/1
  Data Type Conversion/1 -> Simulink-PS Converter1/1
  connections:
  Simulink-PS Converter1/RConn1 -- Ideal Semiconductor Switch/LConn1
  Ideal Semiconductor Switch/RConn1 -- Diode/RConn1 -- +/RConn1
  Ideal Semiconductor Switch/RConn2 -- Diode/LConn1 -- -/RConn1

== system three_phase_solar_grid_SSC/S2 ==
  g : Inport
  Data Type Conversion : DataTypeConversion  SaturateOnIntegerOverflow=off  RndMeth=Floor
  Diode : fl_lib/Electrical/Electrical Elements/Diode  Vf=1e-3 V  Ron=0.01 Ohm  Goff=1e-5 1/Ohm  i_specify=off  i_priority=None  i=0 A  i_nominal_specify=off  i_nominal_value=1  i_nominal_unit=A  v_specify=off  v_priority=None  v=0 V  v_nominal_specify=off  v_nominal_value=1  v_nominal_unit=V
  Ideal Semiconductor Switch : ee_lib/Semiconductors & Converters/Ideal Semiconductor Switch  port_option=ee.enum.controlport.ps  Ron=0.1 Ohm  Goff=1e-5 1/Ohm  Vth=0.5 V  diode_param=ee.enum.semiconductors.protectionDiode.external  diode_Vf=1e-3 V  diode_Ron=0.01 Ohm  diode_Goff=1e-5 1/Ohm  diode_C=50e-9 F  diode_iRM=-235 A  diode_iF=300 A  diode_idot=-50 A/us  diode_trr_param=ee.enum.converters.diodetrr.trr_factor  diode_trr_factor=3  diode_trr=15 us  diode_Qrr=1500 s*uA
  Simulink-PS Converter1 : nesl_utility/Simulink-PS Converter  PhysicalDomain=network_engine_domain  SubClassName=ps_input  LeftPortType=input  RightPortType=output  PseudoPeriodic=off  Frequencies=[]  NoiseDistribution=none  NoiseParameters=[]  Unit=1  AffineConversion=off  FilteringAndDerivatives=provide  SimscapeFilterOrder=1  InputFilterTimeConstant=0.001  UdotUserProvided=0
  + : PMIOPort  Side=Left
  - : PMIOPort  Port=2  Side=Right
  wires:
  Data Type Conversion/1 -> Simulink-PS Converter1/1
  g/1 -> Data Type Conversion/1
  connections:
  Diode/LConn1 -- Ideal Semiconductor Switch/RConn2 -- -/RConn1
  Diode/RConn1 -- Ideal Semiconductor Switch/RConn1 -- +/RConn1
  Simulink-PS Converter1/RConn1 -- Ideal Semiconductor Switch/LConn1

== system three_phase_solar_grid_SSC/S3 ==
  g : Inport
  Data Type Conversion : DataTypeConversion  SaturateOnIntegerOverflow=off  RndMeth=Floor
  Diode : fl_lib/Electrical/Electrical Elements/Diode  Vf=1e-3 V  Ron=0.01 Ohm  Goff=1e-5 1/Ohm  i_specify=off  i_priority=None  i=0 A  i_nominal_specify=off  i_nominal_value=1  i_nominal_unit=A  v_specify=off  v_priority=None  v=0 V  v_nominal_specify=off  v_nominal_value=1  v_nominal_unit=V
  Ideal Semiconductor Switch : ee_lib/Semiconductors & Converters/Ideal Semiconductor Switch  port_option=ee.enum.controlport.ps  Ron=0.1 Ohm  Goff=1e-5 1/Ohm  Vth=0.5 V  diode_param=ee.enum.semiconductors.protectionDiode.external  diode_Vf=1e-3 V  diode_Ron=0.01 Ohm  diode_Goff=1e-5 1/Ohm  diode_C=50e-9 F  diode_iRM=-235 A  diode_iF=300 A  diode_idot=-50 A/us  diode_trr_param=ee.enum.converters.diodetrr.trr_factor  diode_trr_factor=3  diode_trr=15 us  diode_Qrr=1500 s*uA
  Simulink-PS Converter1 : nesl_utility/Simulink-PS Converter  PhysicalDomain=network_engine_domain  SubClassName=ps_input  LeftPortType=input  RightPortType=output  PseudoPeriodic=off  Frequencies=[]  NoiseDistribution=none  NoiseParameters=[]  Unit=1  AffineConversion=off  FilteringAndDerivatives=provide  SimscapeFilterOrder=1  InputFilterTimeConstant=0.001  UdotUserProvided=0
  + : PMIOPort  Side=Left
  - : PMIOPort  Port=2  Side=Right
  wires:
  Data Type Conversion/1 -> Simulink-PS Converter1/1
  g/1 -> Data Type Conversion/1
  connections:
  Diode/LConn1 -- Ideal Semiconductor Switch/RConn2 -- -/RConn1
  Diode/RConn1 -- Ideal Semiconductor Switch/RConn1 -- +/RConn1
  Simulink-PS Converter1/RConn1 -- Ideal Semiconductor Switch/LConn1

== system three_phase_solar_grid_SSC/S4 ==
  g : Inport
  Data Type Conversion : DataTypeConversion  SaturateOnIntegerOverflow=off  RndMeth=Floor
  Diode : fl_lib/Electrical/Electrical Elements/Diode  Vf=1e-3 V  Ron=0.01 Ohm  Goff=1e-5 1/Ohm  i_specify=off  i_priority=None  i=0 A  i_nominal_specify=off  i_nominal_value=1  i_nominal_unit=A  v_specify=off  v_priority=None  v=0 V  v_nominal_specify=off  v_nominal_value=1  v_nominal_unit=V
  Ideal Semiconductor Switch : ee_lib/Semiconductors & Converters/Ideal Semiconductor Switch  port_option=ee.enum.controlport.ps  Ron=0.1 Ohm  Goff=1e-5 1/Ohm  Vth=0.5 V  diode_param=ee.enum.semiconductors.protectionDiode.external  diode_Vf=1e-3 V  diode_Ron=0.01 Ohm  diode_Goff=1e-5 1/Ohm  diode_C=50e-9 F  diode_iRM=-235 A  diode_iF=300 A  diode_idot=-50 A/us  diode_trr_param=ee.enum.converters.diodetrr.trr_factor  diode_trr_factor=3  diode_trr=15 us  diode_Qrr=1500 s*uA
  Simulink-PS Converter1 : nesl_utility/Simulink-PS Converter  PhysicalDomain=network_engine_domain  SubClassName=ps_input  LeftPortType=input  RightPortType=output  PseudoPeriodic=off  Frequencies=[]  NoiseDistribution=none  NoiseParameters=[]  Unit=1  AffineConversion=off  FilteringAndDerivatives=provide  SimscapeFilterOrder=1  InputFilterTimeConstant=0.001  UdotUserProvided=0
  + : PMIOPort  Side=Left
  - : PMIOPort  Port=2  Side=Right
  wires:
  g/1 -> Data Type Conversion/1
  Data Type Conversion/1 -> Simulink-PS Converter1/1
  connections:
  Simulink-PS Converter1/RConn1 -- Ideal Semiconductor Switch/LConn1
  +/RConn1 -- Ideal Semiconductor Switch/RConn1 -- Diode/RConn1
  -/RConn1 -- Ideal Semiconductor Switch/RConn2 -- Diode/LConn1

== system three_phase_solar_grid_SSC/S5 ==
  g : Inport
  Data Type Conversion : DataTypeConversion  SaturateOnIntegerOverflow=off  RndMeth=Floor
  Diode : fl_lib/Electrical/Electrical Elements/Diode  Vf=1e-3 V  Ron=0.01 Ohm  Goff=1e-5 1/Ohm  i_specify=off  i_priority=None  i=0 A  i_nominal_specify=off  i_nominal_value=1  i_nominal_unit=A  v_specify=off  v_priority=None  v=0 V  v_nominal_specify=off  v_nominal_value=1  v_nominal_unit=V
  Ideal Semiconductor Switch : ee_lib/Semiconductors & Converters/Ideal Semiconductor Switch  port_option=ee.enum.controlport.ps  Ron=0.1 Ohm  Goff=1e-5 1/Ohm  Vth=0.5 V  diode_param=ee.enum.semiconductors.protectionDiode.external  diode_Vf=1e-3 V  diode_Ron=0.01 Ohm  diode_Goff=1e-5 1/Ohm  diode_C=50e-9 F  diode_iRM=-235 A  diode_iF=300 A  diode_idot=-50 A/us  diode_trr_param=ee.enum.converters.diodetrr.trr_factor  diode_trr_factor=3  diode_trr=15 us  diode_Qrr=1500 s*uA
  Simulink-PS Converter1 : nesl_utility/Simulink-PS Converter  PhysicalDomain=network_engine_domain  SubClassName=ps_input  LeftPortType=input  RightPortType=output  PseudoPeriodic=off  Frequencies=[]  NoiseDistribution=none  NoiseParameters=[]  Unit=1  AffineConversion=off  FilteringAndDerivatives=provide  SimscapeFilterOrder=1  InputFilterTimeConstant=0.001  UdotUserProvided=0
  + : PMIOPort  Side=Left
  - : PMIOPort  Port=2  Side=Right
  wires:
  g/1 -> Data Type Conversion/1
  Data Type Conversion/1 -> Simulink-PS Converter1/1
  connections:
  Simulink-PS Converter1/RConn1 -- Ideal Semiconductor Switch/LConn1
  +/RConn1 -- Ideal Semiconductor Switch/RConn1 -- Diode/RConn1
  -/RConn1 -- Ideal Semiconductor Switch/RConn2 -- Diode/LConn1

== system three_phase_solar_grid_SSC/S6 ==
  g : Inport
  Data Type Conversion : DataTypeConversion  SaturateOnIntegerOverflow=off  RndMeth=Floor
  Diode : fl_lib/Electrical/Electrical Elements/Diode  Vf=1e-3 V  Ron=0.01 Ohm  Goff=1e-5 1/Ohm  i_specify=off  i_priority=None  i=0 A  i_nominal_specify=off  i_nominal_value=1  i_nominal_unit=A  v_specify=off  v_priority=None  v=0 V  v_nominal_specify=off  v_nominal_value=1  v_nominal_unit=V
  Ideal Semiconductor Switch : ee_lib/Semiconductors & Converters/Ideal Semiconductor Switch  port_option=ee.enum.controlport.ps  Ron=0.1 Ohm  Goff=1e-5 1/Ohm  Vth=0.5 V  diode_param=ee.enum.semiconductors.protectionDiode.external  diode_Vf=1e-3 V  diode_Ron=0.01 Ohm  diode_Goff=1e-5 1/Ohm  diode_C=50e-9 F  diode_iRM=-235 A  diode_iF=300 A  diode_idot=-50 A/us  diode_trr_param=ee.enum.converters.diodetrr.trr_factor  diode_trr_factor=3  diode_trr=15 us  diode_Qrr=1500 s*uA
  Simulink-PS Converter1 : nesl_utility/Simulink-PS Converter  PhysicalDomain=network_engine_domain  SubClassName=ps_input  LeftPortType=input  RightPortType=output  PseudoPeriodic=off  Frequencies=[]  NoiseDistribution=none  NoiseParameters=[]  Unit=1  AffineConversion=off  FilteringAndDerivatives=provide  SimscapeFilterOrder=1  InputFilterTimeConstant=0.001  UdotUserProvided=0
  + : PMIOPort  Side=Left
  - : PMIOPort  Port=2  Side=Right
  wires:
  Data Type Conversion/1 -> Simulink-PS Converter1/1
  g/1 -> Data Type Conversion/1
  connections:
  Diode/LConn1 -- Ideal Semiconductor Switch/RConn2 -- -/RConn1
  Diode/RConn1 -- Ideal Semiconductor Switch/RConn1 -- +/RConn1
  Simulink-PS Converter1/RConn1 -- Ideal Semiconductor Switch/LConn1

== system three_phase_solar_grid_SSC/Subsystem ==
  Phase Splitter1 : ee_lib/Connectors & References/Phase Splitter
  ~ : PMIOPort  Side=Left
  connections:
  Phase Splitter1/RConn1 -- Phase Splitter1/RConn2 -- Phase Splitter1/RConn3
  ~/RConn1 -- Phase Splitter1/LConn1

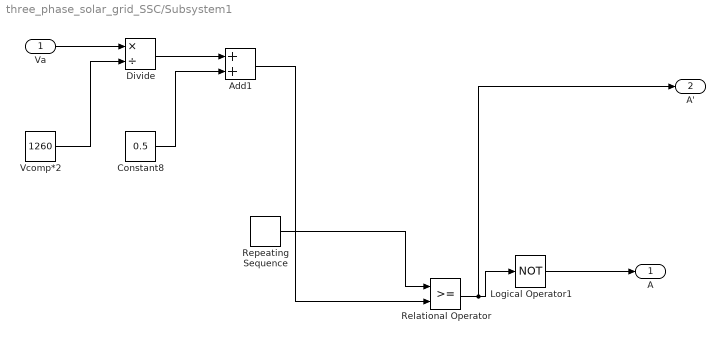
== system three_phase_solar_grid_SSC/Subsystem1 ==
  Va : Inport
  Add1 : Sum
  Constant8 : Constant  Value=0.5
  Divide : Product  Inputs=*/
  Logical Operator1 : Logic  Operator=NOT  AllPortsSameDT=off  OutDataTypeStr=boolean
  Relational Operator : RelationalOperator  OutDataTypeStr=boolean  ZeroCross=off  InputSameDT=off
  Repeating Sequence : simulink/Sources/Repeating Sequence  rep_seq_t=[0 1/100000/2 1/100000]  rep_seq_y=[0 1 0]
  Vcomp*2 : Constant  Value=1260
  A : Outport
  A' : Outport  Port=2
  wires:
  Va/1 -> Divide/1
  Divide/1 -> Add1/1
  Add1/1 -> Relational Operator/2
  Constant8/1 -> Add1/2
  Repeating Sequence/1 -> Relational Operator/1
  Logical Operator1/1 -> A/1
  Relational Operator/1 -> A'/1, Logical Operator1/1
  Vcomp*2/1 -> Divide/2

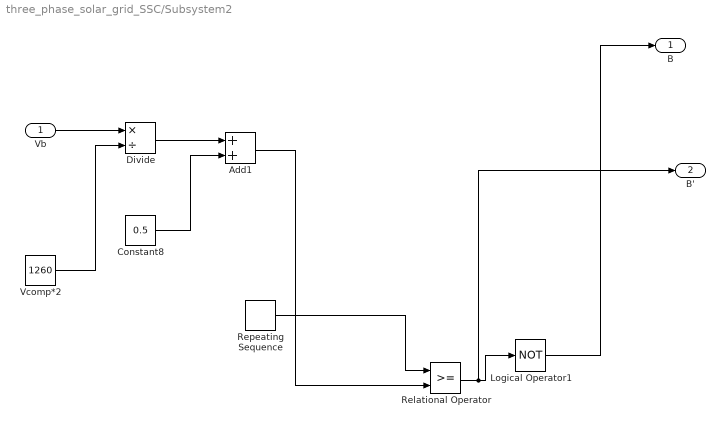
== system three_phase_solar_grid_SSC/Subsystem2 ==
  Vb : Inport
  Add1 : Sum
  Constant8 : Constant  Value=0.5
  Divide : Product  Inputs=*/
  Logical Operator1 : Logic  Operator=NOT  AllPortsSameDT=off  OutDataTypeStr=boolean
  Relational Operator : RelationalOperator  OutDataTypeStr=boolean  ZeroCross=off  InputSameDT=off
  Repeating Sequence : simulink/Sources/Repeating Sequence  rep_seq_t=[0 1/100000/2 1/100000]  rep_seq_y=[0 1 0]
  Vcomp*2 : Constant  Value=1260
  B : Outport
  B' : Outport  Port=2
  wires:
  Vb/1 -> Divide/1
  Divide/1 -> Add1/1
  Add1/1 -> Relational Operator/2
  Constant8/1 -> Add1/2
  Repeating Sequence/1 -> Relational Operator/1
  Logical Operator1/1 -> B/1
  Relational Operator/1 -> B'/1, Logical Operator1/1
  Vcomp*2/1 -> Divide/2

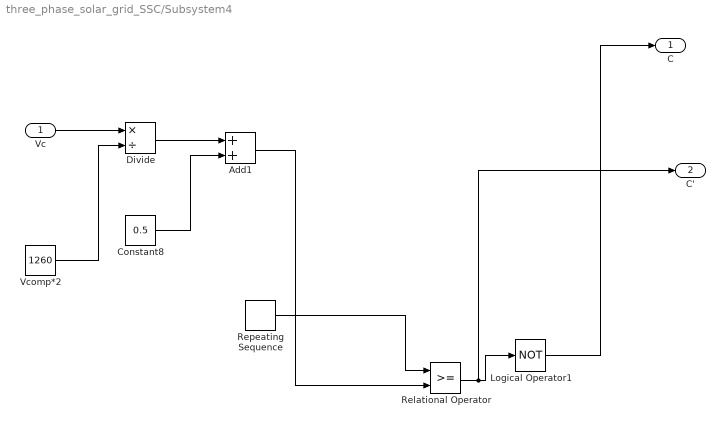
== system three_phase_solar_grid_SSC/Subsystem4 ==
  Vc : Inport
  Add1 : Sum
  Constant8 : Constant  Value=0.5
  Divide : Product  Inputs=*/
  Logical Operator1 : Logic  Operator=NOT  AllPortsSameDT=off  OutDataTypeStr=boolean
  Relational Operator : RelationalOperator  OutDataTypeStr=boolean  ZeroCross=off  InputSameDT=off
  Repeating Sequence : simulink/Sources/Repeating Sequence  rep_seq_t=[0 1/100000/2 1/100000]  rep_seq_y=[0 1 0]
  Vcomp*2 : Constant  Value=1260
  C : Outport
  C' : Outport  Port=2
  wires:
  Vc/1 -> Divide/1
  Divide/1 -> Add1/1
  Add1/1 -> Relational Operator/2
  Constant8/1 -> Add1/2
  Repeating Sequence/1 -> Relational Operator/1
  Logical Operator1/1 -> C/1
  Relational Operator/1 -> C'/1, Logical Operator1/1
  Vcomp*2/1 -> Divide/2

== system three_phase_solar_grid_SSC/curr meas ==
  Current Sensor : fl_lib/Electrical/Electrical Sensors/Current Sensor
  PS-Simulink Converter : nesl_utility/PS-Simulink Converter  PhysicalDomain=network_engine_domain  SubClassName=ps_output  LeftPortType=input  RightPortType=output  PseudoPeriodic=off  Frequencies=[]  VectorFormat=inherit  Unit=inherit  AffineConversion=off
  + : PMIOPort  Side=Left
  - : PMIOPort  Port=2  Side=Right
  I : Outport
  wires:
  PS-Simulink Converter/1 -> I/1
  connections:
  Current Sensor/RConn2 -- -/RConn1
  Current Sensor/LConn1 -- +/RConn1
  PS-Simulink Converter/LConn1 -- Current Sensor/RConn1

== system three_phase_solar_grid_SSC/curr meas (3ph) ==
  Current Sensor (Three-Phase) : ee_lib/Sensors & Transducers/Current Sensor (Three-Phase)
  PS-Simulink Converter : nesl_utility/PS-Simulink Converter  PhysicalDomain=network_engine_domain  SubClassName=ps_output  LeftPortType=input  RightPortType=output  PseudoPeriodic=off  Frequencies=[]  VectorFormat=inherit  Unit=inherit  AffineConversion=off
  ~1 : PMIOPort  Side=Left
  ~2 : PMIOPort  Port=2  Side=Right
  I : Outport
  wires:
  PS-Simulink Converter/1 -> I/1
  connections:
  PS-Simulink Converter/LConn1 -- Current Sensor (Three-Phase)/RConn1
  Current Sensor (Three-Phase)/LConn1 -- ~1/RConn1
  Current Sensor (Three-Phase)/RConn2 -- ~2/RConn1

== system three_phase_solar_grid_SSC/volt meas1 ==
  PS-Simulink Converter1 : nesl_utility/PS-Simulink Converter  PhysicalDomain=network_engine_domain  SubClassName=ps_output  LeftPortType=input  RightPortType=output  PseudoPeriodic=off  Frequencies=[]  VectorFormat=inherit  Unit=inherit  AffineConversion=off
  Voltage Sensor : fl_lib/Electrical/Electrical Sensors/Voltage Sensor
  + : PMIOPort  Side=Left
  - : PMIOPort  Port=2  Side=Right
  V : Outport
  wires:
  PS-Simulink Converter1/1 -> V/1
  connections:
  PS-Simulink Converter1/LConn1 -- Voltage Sensor/RConn1
  Voltage Sensor/RConn2 -- -/RConn1
  Voltage Sensor/LConn1 -- +/RConn1

== matlab function three_phase_solar_grid_SSC/MATLAB Function ==
  data: irradiance output; t input
function irradiance     =   init(t)

if t<0.3
    irradiance=1000;
    
elseif t<0.5
    irradiance=800;
    
else
   irradiance=1000;

end
